simulink model "mec2_dcmotor_loadchange"  (R2018b)
settings: Solver=VariableStepAuto  StartTime=0.0  StopTime=10  MaxStep=1e-2  RelTol=1e-3  AbsTol=1e-3  EnableMultiTasking=on
libraries: fl_lib x34, nesl_utility x15
CloseFcn:
  | try,close(h1_ssc_dcmotor),end
  | clear h1_ssc_dcmotor
  | 
  | clear simlog_ssc_dcmotor
Description:
  | Permanent Magnet DC Motor
  | 
  | Copyright 2008-2018 The MathWorks, Inc.
settings Model: Creator=MathWorks  LastModifiedBy=Latte
settings SolverCC: AutoScaleAbsTol=off
settings DataIOCC: LimitDataPoints=on  SaveFormat=Array
settings OptimizationCC: LifeSpan=inf
settings DebuggingCC: SolverPrmCheckMsg=warning  AllowSymbolicDim=off  LibraryContextMissingDiagnostic=none  SFUnexpectedBacktrackingDiag=warning  SFNoUnconditionalDefaultTransitionDiag=warning  SFExecutionAtInitializationDiag=none
settings HardwareCC: ProdBitPerPointer=32  ProdBitPerSizeT=32  ProdBitPerPtrDiffT=32  ProdLargestAtomicFloat=None  ProdIntDivRoundTo=Undefined  ProdEndianess=Unspecified  ProdWordSize=32  ProdHWDeviceType=32-bit Generic
settings ModelReferenceCC: PropagateSignalLabelsOutOfModel=off
settings SFSimCC: SimUseLocalCustomCode=off
settings RTWCC: RTWUseLocalCustomCode=off
settings CodeAppCC: StateflowObjectComments=on
settings GRTTargetCC: TargetLangStandard=C89/C90 (ANSI)  GeneratePreprocessorConditionals=Disable all
settings ConfigComp: CovMetricSettings=dw  CovHtmlReporting=on  CovSaveCumulativeToWorkspaceVar=on  CovSaveSingleToWorkspaceVar=on  CovExternalEMLEnable=off  CovSFcnEnable=off
settings SimscapeCC: SimscapeLogType=all  SimscapeLogSimulationStatistics=on  SimscapeLogName=simlog_mec2_dcmotor  SimscapeLogDataHistory=10000

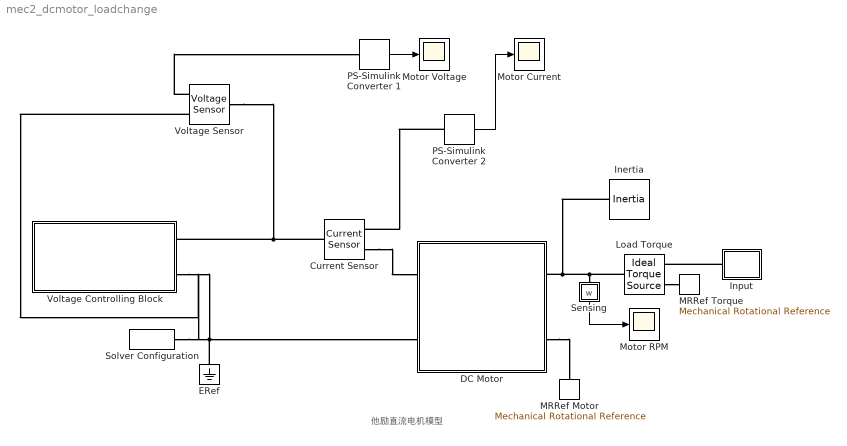
== system mec2_dcmotor_loadchange ==
  note: 他励直流电机模型
  Current Sensor : fl_lib/Electrical/Electrical Sensors/Current Sensor
  DC Motor : Subsystem  Tag=PublishSubsystem
      mask Display:
      | % Circle, in/out, and 'M'
      | image(imread('ssc_dcmotor_maskicon.png'));
      | 
      | % % Circle
      | % plot(sin(0:0.1:2.2*pi)*0.9,cos(0:0.1:2.2*pi)*0.9);
      | %
      | % % In/out
      | % plot([-1.3 -0.9],[0 0]);
      | % plot([1.3 0.9],[0 0]);
      | %
      | % % 'M'
      | % plot([0.5 0.5],[-0.5 0.5]);
      | % plot([-0.5 -0.5],[-0.5 0.5]);
      | % plot([0.5 0],[0.5 -0.5]);
      | % plot([-0.5 0],[0.5 -0.5]);
      | 
      | % Plot points to set plot range
      | color('white');plot(1.5,1.5);plot(-1.5,-1.5)
      | color('black');
      | 
      | port_label('RConn',1,'R');
      | port_label('RConn',2,'C');
      | port_label('LConn',1,'V+');
      | port_label('LConn',2,'V-');
  ERef : fl_lib/Electrical/Electrical Elements/Electrical Reference
  Inertia : fl_lib/Mechanical/Rotational Elements/Inertia  inertia=10 kg*m^2  w_specify=off  w_priority=High  w=0 rad/s  w_nominal_specify=off  w_nominal_unit=rad/s  w_nominal_value=1  t_specify=off  t_priority=None  t=0 N*m  t_nominal_specify=off  t_nominal_unit=N*m  t_nominal_value=1
  Input : Subsystem
  Load Torque : fl_lib/Mechanical/Mechanical Sources/Ideal Torque Source
  MRRef Motor : fl_lib/Mechanical/Rotational Elements/Mechanical Rotational Reference
  MRRef Torque : fl_lib/Mechanical/Rotational Elements/Mechanical Rotational Reference
  Motor Current : Scope
  Motor RPM : Scope
  Motor Voltage : Scope
  PS-Simulink Converter 1 : nesl_utility/PS-Simulink Converter  PhysicalDomain=network_engine_domain  SubClassName=ps_output  LeftPortType=input  RightPortType=output  PseudoPeriodic=off  Frequencies=[]  Unit=V  AffineConversion=on
  PS-Simulink Converter 2 : nesl_utility/PS-Simulink Converter  PhysicalDomain=network_engine_domain  SubClassName=ps_output  LeftPortType=input  RightPortType=output  PseudoPeriodic=off  Frequencies=[]  Unit=A  AffineConversion=off
  Sensing : Subsystem
      mask Display: disp('w');
  Solver Configuration : nesl_utility/Solver Configuration  PhysicalDomain=network_engine_domain  SubClassName=solver  LeftPortType=input  RightPortType=generic  Tones=[]  Harmonics=[]  SimulateNoise=off  Profile=off  UseLocalSampling=off  EnableSwitchedLinearOptims=on  FrequencyDomain=off  UseCCode=off  RelTol=0.001  AbsTol=1e-06  MinStep=1e-09  ToWorkspace=off  RevertToSquareIcSolve=off  NumHomotopyIterations=100  PhasorMode=off  PhasorModeNumHarmonics=1  DoDC=off  ResidualTolerance=1e-9  UseLocalSolver=off  LocalSolverChoice=NE_BACKWARD_EULER_ADVANCER  LocalSolverSampleTime=.001  DoFixedCost=off  MaxNonlinIter=3  MaxModeIter=2  LinearAlgebra=auto  EquationFormulation=NE_TIME_EF  DelaysMemoryBudget=1024  AutomaticFiltering=on  FilteringTimeConstant=0.001  PartitionStorageMethod=AS_NEEDED  PartitionMemoryBudget=1024
  Voltage Controlling Block : Subsystem
  Voltage Sensor : fl_lib/Electrical/Electrical Sensors/Voltage Sensor
  wires:
  Sensing/1(w) -> Motor RPM/1
  PS-Simulink Converter 1/1 -> Motor Voltage/1
  PS-Simulink Converter 2/1 -> Motor Current/1
  connections:
  ERef/LConn1 -- Voltage Sensor/RConn2 -- Voltage Controlling Block/RConn2 -- DC Motor/LConn2 -- Solver Configuration/RConn1
  DC Motor/RConn2 -- MRRef Motor/LConn1
  Load Torque/LConn1 -- Sensing/LConn1 -- Inertia/LConn1 -- DC Motor/RConn1
  Load Torque/RConn2 -- MRRef Torque/LConn1
  Input/LConn1 -- Load Torque/RConn1
  Voltage Sensor/LConn1 -- Voltage Controlling Block/RConn1 -- Current Sensor/LConn1
  Voltage Sensor/RConn1 -- PS-Simulink Converter 1/LConn1
  Current Sensor/RConn2 -- DC Motor/LConn1
  PS-Simulink Converter 2/LConn1 -- Current Sensor/RConn1

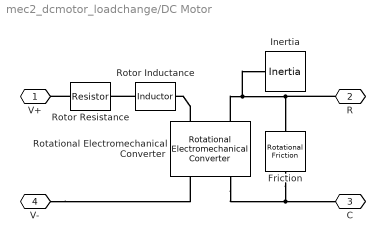
== system mec2_dcmotor_loadchange/DC Motor ==
  Friction : fl_lib/Mechanical/Rotational Elements/Rotational Friction  brkwy_trq=0.02e-3 N*m  brkwy_vel=0.03347 rad/s  Col_trq=0.02e-3 N*m  visc_coef=0.117 N*m/(rad/s)  w_specify=off  w_priority=High  w=0 rad/s  w_nominal_specify=off  w_nominal_unit=rad/s  w_nominal_value=1  t_specify=off  t_priority=High  t=0 N*m  t_nominal_specify=off  t_nominal_unit=N*m  t_nominal_value=1
      settings: SourceProductName=Simscape
  Inertia : fl_lib/Mechanical/Rotational Elements/Inertia  inertia=1.82 kg*m^2  w_specify=off  w_priority=High  w=0 rad/s  w_nominal_specify=off  w_nominal_unit=rad/s  w_nominal_value=1  t_specify=off  t_priority=High  t=0 N*m  t_nominal_specify=off  t_nominal_unit=N*m  t_nominal_value=1
  Rotational Electromechanical Converter : fl_lib/Electrical/Electrical Elements/Rotational Electromechanical Converter  K=1.225 V/(rad/s)  i_specify=off  i_priority=High  i=0 A  i_nominal_specify=off  i_nominal_unit=A  i_nominal_value=1  v_specify=off  v_priority=High  v=0 V  v_nominal_specify=off  v_nominal_unit=V  v_nominal_value=1  t_specify=off  t_priority=High  t=0 N*m  t_nominal_specify=off  t_nominal_unit=N*m  t_nominal_value=1  w_specify=off  w_priority=High  w=0 rad/s  w_nominal_specify=off  w_nominal_unit=rad/s  w_nominal_value=1
      settings: SourceProductName=Simscape
  Rotor Inductance : fl_lib/Electrical/Electrical Elements/Inductor  l=11e-4 H  r=0 Ohm  g=0 1/Ohm  i_specify=off  i_priority=High  i=0 A  i_nominal_specify=off  i_nominal_unit=A  i_nominal_value=1  v_specify=off  v_priority=High  v=0 V  v_nominal_specify=off  v_nominal_unit=V  v_nominal_value=1  i_L_specify=on  i_L_priority=High  i_L=0 A  i_L_nominal_specify=off  i_L_nominal_unit=A  i_L_nominal_value=1
  Rotor Resistance : fl_lib/Electrical/Electrical Elements/Resistor  Tag=Factory Generic  R=0.0144 Ohm  i_specify=off  i_priority=High  i=0 A  i_nominal_specify=off  i_nominal_unit=A  i_nominal_value=1  v_specify=off  v_priority=High  v=0 V  v_nominal_specify=off  v_nominal_unit=V  v_nominal_value=1
  V+ : PMIOPort  Side=Left
  R : PMIOPort  Port=2  Side=Right
  C : PMIOPort  Port=3  Side=Right
  V- : PMIOPort  Port=4  Side=Left
  connections:
  Rotational Electromechanical Converter/LConn1 -- Rotor Inductance/RConn1
  V-/RConn1 -- Rotational Electromechanical Converter/RConn1
  Rotor Resistance/LConn1 -- V+/RConn1
  Rotor Inductance/LConn1 -- Rotor Resistance/RConn1
  Rotational Electromechanical Converter/LConn2 -- R/RConn1 -- Friction/LConn1 -- Inertia/LConn1
  Rotational Electromechanical Converter/RConn2 -- C/RConn1 -- Friction/RConn1

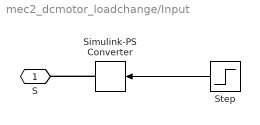
== system mec2_dcmotor_loadchange/Input ==
  Simulink-PS Converter : nesl_utility/Simulink-PS Converter  PhysicalDomain=network_engine_domain  SubClassName=ps_input  LeftPortType=input  RightPortType=output  PseudoPeriodic=off  Frequencies=[]  NoiseDistribution=none  NoiseParameters=[]  Unit=1  AffineConversion=off  FilteringAndDerivatives=zero  SimscapeFilterOrder=1  InputFilterTimeConstant=.001  UdotUserProvided=0
  Step : Step  Time=3  After=-420  SampleTime=0
  S : PMIOPort  Side=Left
  wires:
  Step/1 -> Simulink-PS Converter/1
  connections:
  Simulink-PS Converter/RConn1 -- S/RConn1

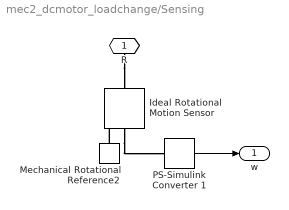
== system mec2_dcmotor_loadchange/Sensing ==
  Ideal Rotational Motion Sensor : fl_lib/Mechanical/Mechanical Sensors/Ideal Rotational Motion Sensor  offset=0 rad
  Mechanical Rotational Reference2 : fl_lib/Mechanical/Rotational Elements/Mechanical Rotational Reference
  PS-Simulink Converter 1 : nesl_utility/PS-Simulink Converter  PhysicalDomain=network_engine_domain  SubClassName=ps_output  LeftPortType=input  RightPortType=output  PseudoPeriodic=off  Frequencies=[]  Unit=rpm  AffineConversion=off
  R : PMIOPort  Side=Left
  w : Outport
  wires:
  PS-Simulink Converter 1/1 -> w/1
  connections:
  Ideal Rotational Motion Sensor/RConn2 -- PS-Simulink Converter 1/LConn1
  Mechanical Rotational Reference2/LConn1 -- Ideal Rotational Motion Sensor/RConn1
  R/RConn1 -- Ideal Rotational Motion Sensor/LConn1

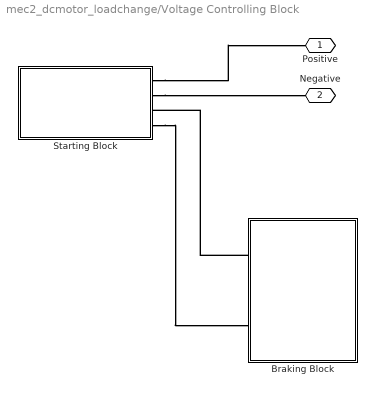
== system mec2_dcmotor_loadchange/Voltage Controlling Block ==
  Braking Block : Subsystem
  Starting Block : Subsystem
  Positive : PMIOPort  Side=Right
  Negative : PMIOPort  Port=2  Side=Right
  connections:
  Starting Block/RConn2 -- Negative/RConn1
  Starting Block/RConn1 -- Positive/RConn1
  Braking Block/LConn1 -- Starting Block/RConn3
  Starting Block/RConn4 -- Braking Block/LConn2

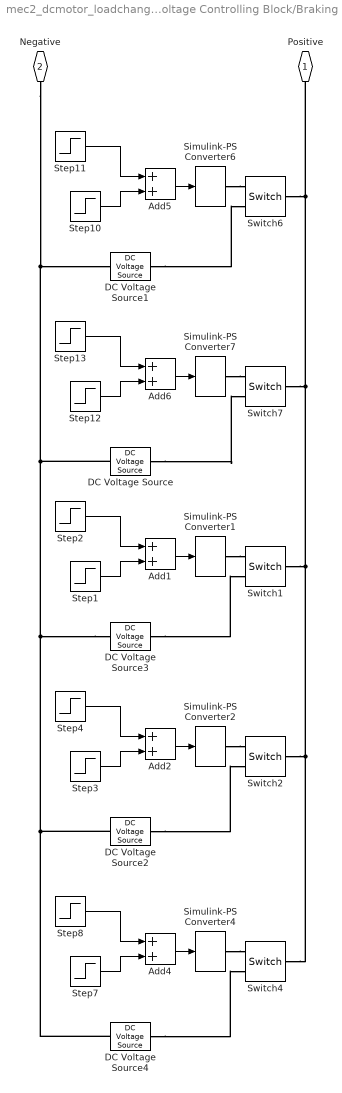
== system mec2_dcmotor_loadchange/Voltage Controlling Block/Braking Block ==
  Add{1..2,4..6} (5 alike) : Sum
  DC Voltage Source : fl_lib/Electrical/Electrical Sources/DC Voltage Source  v0=110 V
  DC Voltage Source1 : fl_lib/Electrical/Electrical Sources/DC Voltage Source  v0=170 V
  DC Voltage Source2 : fl_lib/Electrical/Electrical Sources/DC Voltage Source  v0=8.3 V
  DC Voltage Source3 : fl_lib/Electrical/Electrical Sources/DC Voltage Source  v0=50 V
  DC Voltage Source4 : fl_lib/Electrical/Electrical Sources/DC Voltage Source  v0=4.937 V
  Simulink-PS Converter{1..2,4,6..7} (5 alike) : nesl_utility/Simulink-PS Converter  PhysicalDomain=network_engine_domain  SubClassName=ps_input  LeftPortType=input  RightPortType=output  PseudoPeriodic=off  Frequencies=[]  NoiseDistribution=none  NoiseParameters=[]  Unit=1  AffineConversion=off  FilteringAndDerivatives=zero  SimscapeFilterOrder=1  InputFilterTimeConstant=.001  UdotUserProvided=0
  Step1 : Step  Time=8.9  After=-1  SampleTime=0
  Step10 : Step  Time=8.3  After=-1  SampleTime=0
  Step11 : Step  Time=8  SampleTime=0
  Step12 : Step  Time=8.6  After=-1  SampleTime=0
  Step13 : Step  Time=8.3  SampleTime=0
  Step2 : Step  Time=8.6  SampleTime=0
  Step3 : Step  Time=9.23  After=-1  SampleTime=0
  Step4 : Step  Time=8.9  SampleTime=0
  Step7 : Step  Time=20  After=-1  SampleTime=0
  Step8 : Step  Time=9.23  SampleTime=0
  Switch{1..2,4,6..7} (5 alike) : fl_lib/Electrical/Electrical Elements/Switch  R_closed=1e-10 Ohm  G_open=1e-8 1/Ohm  Threshold=0.5  i_specify=off  i_priority=None  i=0 A  i_nominal_specify=off  i_nominal_unit=A  i_nominal_value=1  v_specify=off  v_priority=None  v=0 V  v_nominal_specify=off  v_nominal_unit=V  v_nominal_value=1
      settings: SourceProductName=Simscape
  Positive : PMIOPort  Side=Left
  Negative : PMIOPort  Port=2  Side=Left
  wires:
  Step12/1 -> Add6/2
  Step10/1 -> Add5/2
  Step11/1 -> Add5/1
  Add5/1 -> Simulink-PS Converter6/1
  Add6/1 -> Simulink-PS Converter7/1
  Step13/1 -> Add6/1
  Step4/1 -> Add2/1
  Add1/1 -> Simulink-PS Converter1/1
  Step2/1 -> Add1/1
  Add2/1 -> Simulink-PS Converter2/1
  Step1/1 -> Add1/2
  Step3/1 -> Add2/2
  Step8/1 -> Add4/1
  Add4/1 -> Simulink-PS Converter4/1
  Step7/1 -> Add4/2
  connections:
  Simulink-PS Converter6/RConn1 -- Switch6/RConn1
  DC Voltage Source3/RConn1 -- DC Voltage Source4/RConn1 -- DC Voltage Source2/RConn1 -- Negative/RConn1 -- DC Voltage Source1/RConn1 -- DC Voltage Source/RConn1
  Simulink-PS Converter7/RConn1 -- Switch7/RConn1
  Switch1/LConn1 -- Switch4/LConn1 -- Switch2/LConn1 -- Positive/RConn1 -- Switch6/LConn1 -- Switch7/LConn1
  DC Voltage Source1/LConn1 -- Switch6/RConn2
  DC Voltage Source/LConn1 -- Switch7/RConn2
  Simulink-PS Converter1/RConn1 -- Switch1/RConn1
  DC Voltage Source2/LConn1 -- Switch2/RConn2
  DC Voltage Source3/LConn1 -- Switch1/RConn2
  Simulink-PS Converter2/RConn1 -- Switch2/RConn1
  DC Voltage Source4/LConn1 -- Switch4/RConn2
  Simulink-PS Converter4/RConn1 -- Switch4/RConn1

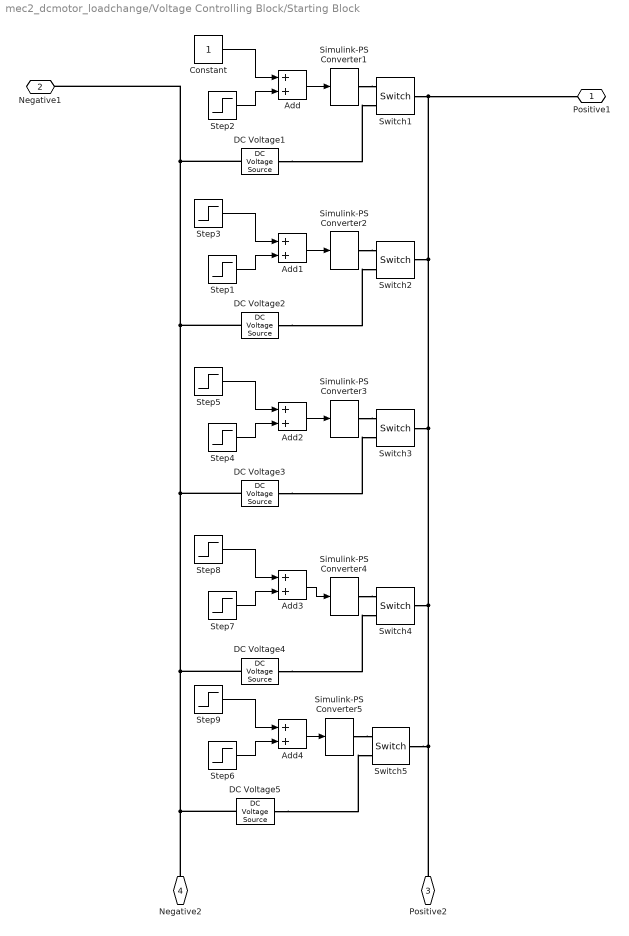
== system mec2_dcmotor_loadchange/Voltage Controlling Block/Starting Block ==
  Add{,1..4} (5 alike) : Sum
  Constant : Constant
  DC Voltage1 : fl_lib/Electrical/Electrical Sources/DC Voltage Source  v0=50 V
  DC Voltage2 : fl_lib/Electrical/Electrical Sources/DC Voltage Source  v0=100 V
  DC Voltage3 : fl_lib/Electrical/Electrical Sources/DC Voltage Source  v0=150 V
  DC Voltage4 : fl_lib/Electrical/Electrical Sources/DC Voltage Source  v0=200 V
  DC Voltage5 : fl_lib/Electrical/Electrical Sources/DC Voltage Source  v0=230 V
  Simulink-PS Converter{1..5} (5 alike) : nesl_utility/Simulink-PS Converter  PhysicalDomain=network_engine_domain  SubClassName=ps_input  LeftPortType=input  RightPortType=output  PseudoPeriodic=off  Frequencies=[]  NoiseDistribution=none  NoiseParameters=[]  Unit=1  AffineConversion=off  FilteringAndDerivatives=zero  SimscapeFilterOrder=1  InputFilterTimeConstant=.001  UdotUserProvided=0
  Step1 : Step  Time=0.6  After=-1  SampleTime=0
  Step2 : Step  Time=0.3  After=-1  SampleTime=0
  Step3 : Step  Time=0.3  SampleTime=0
  Step4 : Step  Time=0.9  After=-1  SampleTime=0
  Step5 : Step  Time=0.6  SampleTime=0
  Step6 : Step  Time=8  After=-1  SampleTime=0
  Step7 : Step  Time=1.2  After=-1  SampleTime=0
  Step8 : Step  Time=0.9  SampleTime=0
  Step9 : Step  Time=1.2  SampleTime=0
  Switch{1..5} (5 alike) : fl_lib/Electrical/Electrical Elements/Switch  R_closed=1e-10 Ohm  G_open=1e-8 1/Ohm  Threshold=0.5  i_specify=off  i_priority=None  i=0 A  i_nominal_specify=off  i_nominal_unit=A  i_nominal_value=1  v_specify=off  v_priority=None  v=0 V  v_nominal_specify=off  v_nominal_unit=V  v_nominal_value=1
      settings: SourceProductName=Simscape
  Positive1 : PMIOPort  Side=Right
  Negative1 : PMIOPort  Port=2  Side=Right
  Positive2 : PMIOPort  Port=3  Side=Right
  Negative2 : PMIOPort  Port=4  Side=Right
  wires:
  Add4/1 -> Simulink-PS Converter5/1
  Step7/1 -> Add3/2
  Add3/1 -> Simulink-PS Converter4/1
  Add/1 -> Simulink-PS Converter1/1
  Step8/1 -> Add3/1
  Step1/1 -> Add1/2
  Step3/1 -> Add1/1
  Add1/1 -> Simulink-PS Converter2/1
  Step9/1 -> Add4/1
  Add2/1 -> Simulink-PS Converter3/1
  Step4/1 -> Add2/2
  Constant/1 -> Add/1
  Step5/1 -> Add2/1
  Step6/1 -> Add4/2
  Step2/1 -> Add/2
  connections:
  Simulink-PS Converter1/RConn1 -- Switch1/RConn1
  Switch1/LConn1 -- Positive1/RConn1 -- Switch5/LConn1 -- Positive2/RConn1 -- Switch4/LConn1 -- Switch3/LConn1 -- Switch2/LConn1
  DC Voltage4/LConn1 -- Switch4/RConn2
  Simulink-PS Converter4/RConn1 -- Switch4/RConn1
  Simulink-PS Converter3/RConn1 -- Switch3/RConn1
  DC Voltage5/LConn1 -- Switch5/RConn2
  Simulink-PS Converter5/RConn1 -- Switch5/RConn1
  DC Voltage1/RConn1 -- Negative1/RConn1 -- Negative2/RConn1 -- DC Voltage5/RConn1 -- DC Voltage4/RConn1 -- DC Voltage3/RConn1 -- DC Voltage2/RConn1
  DC Voltage3/LConn1 -- Switch3/RConn2
  DC Voltage2/LConn1 -- Switch2/RConn2
  Simulink-PS Converter2/RConn1 -- Switch2/RConn1
  DC Voltage1/LConn1 -- Switch1/RConn2
